simulink model "MOSFET_Dynamic_Model"  (R2023b)
settings: Solver=VariableStepAuto  StartTime=0.0  StopTime=0.5  RelTol=1e-3  AbsTol=1e-3
libraries: fl_lib x12, nesl_utility x5
settings Model: Creator=hp  LastModifiedBy=hp
settings SolverCC: AutoScaleAbsTol=off  AlgebraicLoopSolver=TrustRegion  MaxZcPerStep=1
settings DebuggingCC: UnconnectedInputMsg=warning  UnconnectedOutputMsg=warning  UnconnectedLineMsg=warning  SymbolicDimsDataTypeCodeGenerationDiagnostic=none
settings ModelReferenceCC: EnableRefExpFcnMdlSchedulingChecks=on
settings SFSimCC: CustomCodeUndefinedFunction=UseInterfaceOnly
settings RTWCC: DLArmComputeVersion=19.05
settings SimscapeCC: SimscapeLogType=all  SimscapeLogSimulationStatistics=on  SimscapeLogDataHistory=10000

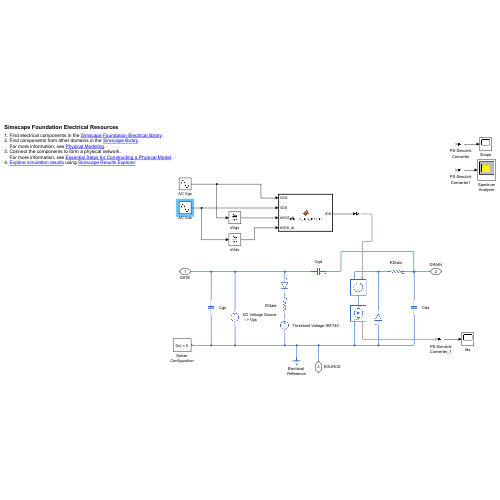
[thumbnail: Simulink's stored preview of the top-level diagram]
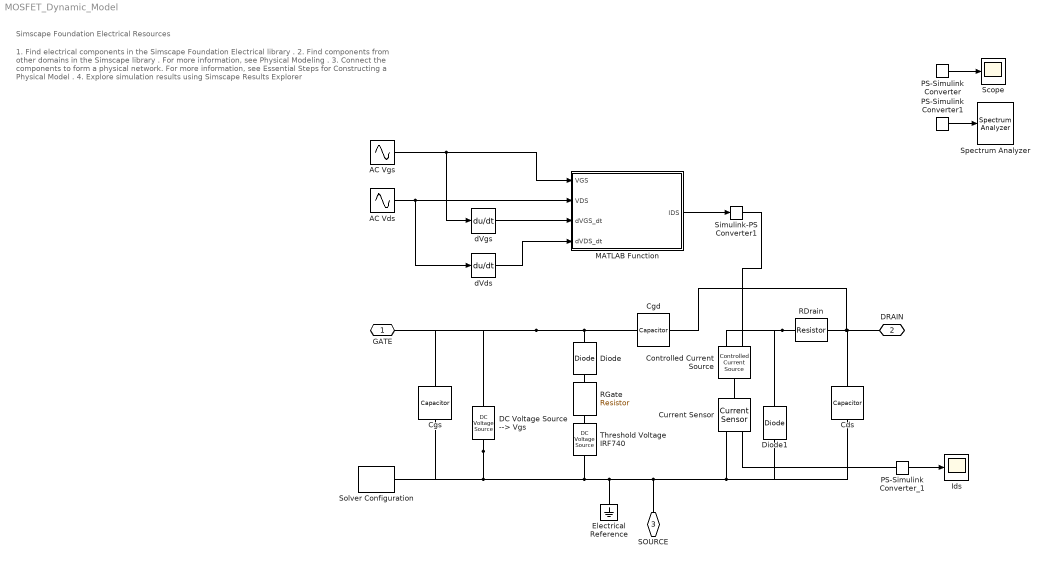
== system MOSFET_Dynamic_Model ==
  note: 1. Find electrical components in the Simscape Foundation Electrical library .
      | 2. Find components from other domains in the Simscape library .
      | For more information, see Physical Modeling .
      | 3. Connect the components to form a physical network.
      | For more information, see Essential Steps for Constructing a Physical Model .
      | 4. Explore simulation results using Simscape Results Explorer
  note: Simscape Foundation Electrical Resources
  AC Vds : Sin  Amplitude=100  Bias=200  Frequency=2*pi*0.8e5  SampleTime=0
  AC Vgs : Sin  Amplitude=10  Frequency=2*pi*0.16e6  SampleTime=0
  Cds : fl_lib/Electrical/Electrical Elements/Capacitor  c=193e-12 F  r=1e-6 Ohm  g=0 1/Ohm  i_specify=off  i_priority=None  i=0 A  i_nominal_specify=off  i_nominal_unit=A  i_nominal_value=1  v_specify=off  v_priority=None  v=0 V  v_nominal_specify=off  v_nominal_unit=V  v_nominal_value=1  vc_specify=off  vc_priority=High  vc=0 V  vc_nominal_specify=off  vc_nominal_unit=V  vc_nominal_value=1
  Cgd : fl_lib/Electrical/Electrical Elements/Capacitor  c=27e-12 F  r=1e-6 Ohm  g=0 1/Ohm  i_specify=off  i_priority=None  i=0 A  i_nominal_specify=off  i_nominal_unit=A  i_nominal_value=1  v_specify=off  v_priority=None  v=0 V  v_nominal_specify=off  v_nominal_unit=V  v_nominal_value=1  vc_specify=off  vc_priority=High  vc=0 V  vc_nominal_specify=off  vc_nominal_unit=V  vc_nominal_value=1
  Cgs : fl_lib/Electrical/Electrical Elements/Capacitor  c=1373e-12 F  r=1e-6 Ohm  g=0 1/Ohm  i_specify=off  i_priority=None  i=0 A  i_nominal_specify=off  i_nominal_unit=A  i_nominal_value=1  v_specify=off  v_priority=None  v=0 V  v_nominal_specify=off  v_nominal_unit=V  v_nominal_value=1  vc_specify=off  vc_priority=High  vc=0 V  vc_nominal_specify=off  vc_nominal_unit=V  vc_nominal_value=1
  Controlled Current Source : fl_lib/Electrical/Electrical Sources/Controlled Current Source
  Current Sensor : fl_lib/Electrical/Electrical Sensors/Current Sensor
  DC Voltage Source --> Vgs : fl_lib/Electrical/Electrical Sources/DC Voltage Source  v0=10 V
  Diode : fl_lib/Electrical/Electrical Elements/Diode  Vf=0.7 V  Ron=0.3 Ohm  Goff=1e-8 1/Ohm  i_specify=off  i_priority=None  i=0 A  i_nominal_specify=off  i_nominal_unit=A  i_nominal_value=1  v_specify=off  v_priority=None  v=0 V  v_nominal_specify=off  v_nominal_unit=V  v_nominal_value=1
  Diode1 : fl_lib/Electrical/Electrical Elements/Diode  Vf=0.7 V  Ron=0.3 Ohm  Goff=1e-8 1/Ohm  i_specify=off  i_priority=None  i=0 A  i_nominal_specify=off  i_nominal_unit=A  i_nominal_value=1  v_specify=off  v_priority=None  v=0 V  v_nominal_specify=off  v_nominal_unit=V  v_nominal_value=1
  Electrical Reference : fl_lib/Electrical/Electrical Elements/Electrical Reference
  Ids : Scope
  MATLAB Function : MATLAB Function  TreatAsAtomicUnit=on
  PS-Simulink Converter : nesl_utility/PS-Simulink Converter  PhysicalDomain=network_engine_domain  SubClassName=ps_output  LeftPortType=input  RightPortType=output  PseudoPeriodic=off  Frequencies=[]  VectorFormat=inherit  Unit=inherit  AffineConversion=off
  PS-Simulink Converter1 : nesl_utility/PS-Simulink Converter  PhysicalDomain=network_engine_domain  SubClassName=ps_output  LeftPortType=input  RightPortType=output  PseudoPeriodic=off  Frequencies=[]  VectorFormat=inherit  Unit=inherit  AffineConversion=off
  PS-Simulink Converter_1 : nesl_utility/PS-Simulink Converter  PhysicalDomain=network_engine_domain  SubClassName=ps_output  LeftPortType=input  RightPortType=output  PseudoPeriodic=off  Frequencies=[]  VectorFormat=inherit  Unit=inherit  AffineConversion=on
  RDrain : fl_lib/Electrical/Electrical Elements/Resistor  R=0.5 Ohm  i_specify=off  i_priority=None  i=0 A  i_nominal_specify=off  i_nominal_unit=A  i_nominal_value=1  v_specify=off  v_priority=None  v=0 V  v_nominal_specify=off  v_nominal_unit=V  v_nominal_value=1
  RGate : fl_lib/Electrical/Electrical Elements/Resistor  R=200000000 Ohm  i_specify=off  i_priority=None  i=0 A  i_nominal_specify=off  i_nominal_unit=A  i_nominal_value=1  v_specify=off  v_priority=None  v=0 V  v_nominal_specify=off  v_nominal_unit=V  v_nominal_value=1
  Scope : Scope
  Simulink-PS Converter1 : nesl_utility/Simulink-PS Converter  PhysicalDomain=network_engine_domain  SubClassName=ps_input  LeftPortType=input  RightPortType=output  PseudoPeriodic=off  Frequencies=[]  NoiseDistribution=none  NoiseParameters=[]  Unit=1  AffineConversion=off  FilteringAndDerivatives=provide  SimscapeFilterOrder=1  InputFilterTimeConstant=0.001  UdotUserProvided=0
  Solver Configuration : nesl_utility/Solver Configuration  PhysicalDomain=network_engine_domain  SubClassName=solver  LeftPortType=input  RightPortType=generic  Tones=[]  Harmonics=[]  SimulateNoise=off  Profile=off  UseLocalSampling=off  EnableSwitchedLinearOptims=on  FrequencyDomain=off  UseCCode=off  RelTol=0.001  AbsTol=1e-06  MinStep=1e-09  ToWorkspace=off  RevertToSquareIcSolve=off  NumHomotopyIterations=100  PhasorMode=off  PhasorModeNumHarmonics=1  ConsistencySolver=NEWTON_XTOL_AFTER_FTOL  IndexReductionMethod=DerivativeReplacement  DoDC=off  ResidualTolerance=1e-09  ConsistencyTolSource=GLOBAL  ConsistencyAbsTol=0.001  ConsistencyRelTol=0.001  ConsistencyTolFactor=0.001  UseLocalSolver=off  LocalSolverChoice=NE_BACKWARD_EULER_ADVANCER  ResolveIndetEquations=on  FunctionEvalNumThread=1  LocalSolverSampleTime=0.001  DoFixedCost=off  MaxNonlinIter=3  MaxModeIter=2  ComputeImpulses=off  ImpulseIterations=2  LinearAlgebra=auto  LinearAlgebraNumThread=0  EquationFormulation=NE_TIME_EF  DelaysMemoryBudget=1024  AutomaticFiltering=on  FilteringTimeConstant=0.001  PartitionStorageMethod=AS_NEEDED  PartitionMemoryBudget=1024  PartitionMethod=ROBUST  MultibodyUseLocalSolver=off  MultibodyLocalSolverChoice=ODE1  MultibodyLocalSolverSampleTime=0.001
  Spectrum Analyzer : SpectrumAnalyzer  WindowPosition=[368.000000,182.000000,800.000000,500.000000,]  ScopeFrameLocation=window  Method=Welch  SampleRate=10e3  PlotAsTwoSidedSpectrum=off  AxesScalingNumUpdates=10  Span=10e3  StartFrequency=-5e3  StopFrequency=5e3  AveragingMethod=Running  YLimits=[-3603.44492261,-2802.67938425]  ShowGrid=off  SegLen=128
  Threshold Voltage IRF740 : fl_lib/Electrical/Electrical Sources/DC Voltage Source  v0=4.7 V
  dVds : Derivative
  dVgs : Derivative
  GATE : PMIOPort  Description=G  Side=Left
  DRAIN : PMIOPort  Port=2  Side=Left
  SOURCE : PMIOPort  Port=3  Side=Left
  wires:
  PS-Simulink Converter/1 -> Scope/1
  PS-Simulink Converter1/1 -> Spectrum Analyzer/1
  MATLAB Function/1(IDS) -> Simulink-PS Converter1/1
  PS-Simulink Converter_1/1 -> Ids/1
  AC Vgs/1 -> dVgs/1, MATLAB Function/1(VGS)
  AC Vds/1 -> dVds/1, MATLAB Function/2(VDS)
  dVgs/1 -> MATLAB Function/3(dVGS_dt)
  dVds/1 -> MATLAB Function/4(dVDS_dt)
  connections:
  DC Voltage Source --> Vgs/RConn1 -- Cgs/LConn1 -- Solver Configuration/RConn1 -- Cds/LConn1 -- Diode1/LConn1 -- Current Sensor/RConn2 -- SOURCE/RConn1 -- Electrical Reference/LConn1 -- Threshold Voltage IRF740/RConn1
  RDrain/RConn1 -- Diode1/RConn1 -- Controlled Current Source/RConn2
  GATE/RConn1 -- Cgs/RConn1 -- DC Voltage Source --> Vgs/LConn1 -- Cgd/RConn1 -- Diode/LConn1
  PS-Simulink Converter_1/LConn1 -- Current Sensor/RConn1
  Current Sensor/LConn1 -- Controlled Current Source/LConn1
  RDrain/LConn1 -- Cgd/LConn1 -- DRAIN/RConn1 -- Cds/RConn1
  Simulink-PS Converter1/RConn1 -- Controlled Current Source/RConn1
  Diode/RConn1 -- RGate/LConn1
  RGate/RConn1 -- Threshold Voltage IRF740/LConn1

== matlab function MOSFET_Dynamic_Model/MATLAB Function ==
  data: VGS input; IDS output; VDS input; dVGS_dt input; dVDS_dt input
function IDS = mosfet_ids_model(VGS, VDS, dVGS_dt, dVDS_dt)
%#codegen
% Calcola IDS in base a VGS, VDS e le derivate, secondo modello dinamico IRF740

% --- Parametri modello IRF740 ---
Vth = 4.7;               % Tensione di soglia [V]
KPLIN = 2.4;             % Guadagno regione lineare [A/V^2]
KPSAT = 8.84;            % Guadagno regione saturazione [A/V^2]
theta = 0.3;             % Effetto Early

% --- Parametri capacitivi ---
Cgs = 1373e-12;          % [F]
Cgd = 27e-12;            % [F]

% --- Limiti ---
Imax_continua = 10;      % [A]
Imax_impulso  = 40;      % [A]
% Nota: la durata dell’impulso va gestita esternamente in Simulink se necessario

% --- Corrente statica ---
if VGS <= Vth
    IDS_static = 0;
elseif VDS < VGS - Vth
    IDS_static = (KPLIN * ((VGS - Vth) * VDS - ...
                 (0.5 * KPLIN / KPSAT * VDS^2))) / ...
                 (1 + theta * VDS);
else
    VDS_border = VGS - Vth;
    ID_border = (KPLIN * ((VGS - Vth) * VDS_border - ...
                 (0.5 * KPLIN / KPSAT * VDS_border^2))) / ...
                 (1 + theta * VDS_border);
    IDS_static = ID_border * (1 + theta * (VDS - VDS_border));
end

% --- Clipping statico ---
IDS_static = min(IDS_static, Imax_continua);

% --- Termini dinamici (capacità) ---
IDS_dynamic = IDS_static + (Cgs + Cgd) * dVGS_dt - Cgd * dVDS_dt;

% --- Clipping impulsivo (durata da gestire fuori) ---
IDS = min(IDS_dynamic, Imax_impulso);
end
